simulink model "test_validation_gate"  (Simulink 7.6)
settings: Solver=FixedStepDiscrete  StartTime=0.0  StopTime=0  RelTol=1e-3
undefined symbols (not defined in the file): gray, Rec, Scale_Forward_B, Scale_Forward_G, Scale_Forward_H, Scale_Forward_R, Scale_Forward_S, Scale_Forward_V, SDTV
libraries: vipsnks x11, viptextngfix x2, vipconversions x2, vipsrcs x1, viptransforms x1
settings Model: Creator=Thing 1  LastModifiedBy=auvt
settings RTWCC: TargetLang=C++

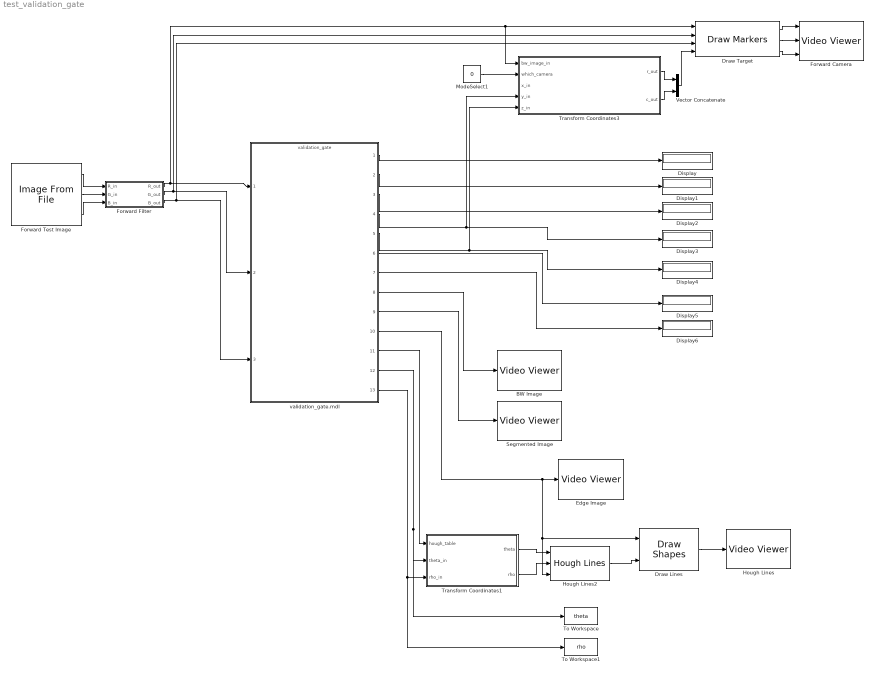
== system test_validation_gate ==
  BW Image : vipsnks/Video Viewer  DialogControllerArgs=DataTag1  inputType=Obsolete7b  imagePorts=One multidimensional signal  useColorMap=off  colormapValue=gray(256)  specRange=off  minInputVal=0  maxInputVal=255  FigPos=[651 667 290 272]  AxisZoom=on  trueSizedOnce=off  OpenAtMdlStart=on
  Display{,1..6} (7 alike) : Display
  Draw Lines : viptextngfix/Draw Shapes  DialogController=vipDDGCreate  DialogControllerArgs=DataTag2  shape=Lines  fill=off  fillClrSource=Specify via dialog  display=User-specified value  intensity=200  color=.5  opacity=0.6  viewport=Entire image  antialiasing=off  inType=Obsolete  imagePorts=One multidimensional signal  prodOutputMode=Binary point scaling  prodOutputWordLength=32  prodOutputFracLength=14  memoryMode=Specify word length  memoryWordLength=16  memoryFracLength=15  roundingMode=Floor  overflowMode=off
  Draw Target : viptextngfix/Draw Markers  DialogController=vipDDGCreate  DialogControllerArgs=DataTag3  shape=X-mark  size=7  fill=off  fillClrSource=Specify via dialog  display=User-specified value  intensity=200  color=[0 0 0]  opacity=0.6  viewport=Entire image  antialiasing=off  inType=Obsolete  imagePorts=Separate color signals  prodOutputMode=Binary point scaling  prodOutputWordLength=32  prodOutputFracLength=14  memoryMode=Specify word length  memoryWordLength=16  memoryFracLength=15  roundingMode=Floor  overflowMode=off
  Edge Image : vipsnks/Video Viewer  DialogControllerArgs=DataTag5  inputType=Obsolete7b  imagePorts=One multidimensional signal  useColorMap=off  colormapValue=gray(256)  specRange=off  minInputVal=0  maxInputVal=255  FigPos=[678 854 521 718]  AxisZoom=on  trueSizedOnce=off  OpenAtMdlStart=on
  Forward Camera : vipsnks/Video Viewer  DialogControllerArgs=DataTag7  inputType=Obsolete7b  imagePorts=Separate color signals  useColorMap=off  colormapValue=gray(256)  specRange=off  minInputVal=0  maxInputVal=255  FigPos=[1001 798 418 649]  AxisZoom=on  trueSizedOnce=off  OpenAtMdlStart=on
  Forward Filter : Subsystem
  Forward Test Image : vipsrcs/Image From File  Tag=vipblks_nd  DialogController=vipDDGCreate  DialogControllerArgs=DataTag20  SystemSampleTime=-1  FileName=/home/auvt/Desktop/Carlo/vlcsnap-2011-06-21-00h16m39s112.png  imagePorts=Separate color signals  Ts=-1  ImageDataType=double  Signed=on  WordLength=16  sdImageDataType=uint(8)  FractionLengthMode=User-defined  FractionLength=15  OutPortLabels=R|G|B
  Hough Lines : vipsnks/Video Viewer  DialogControllerArgs=DataTag22  inputType=Obsolete7b  imagePorts=One multidimensional signal  useColorMap=off  colormapValue=gray(256)  specRange=off  minInputVal=0  maxInputVal=255  FigPos=[-14 868 615 732]  AxisZoom=on  trueSizedOnce=off  OpenAtMdlStart=on
  Hough Lines2 : viptransforms/Hough Lines  DialogController=vipDDGCreate  DialogControllerArgs=DataTag23  sineCompMethod=Trigonometric function  thetaRes=pi/180  firstCoeffMode=Specify word length  firstCoeffWordLength=16  firstCoeffFracLength=15  prodOutputMode=Binary point scaling  prodOutputWordLength=32  prodOutputFracLength=16  roundingMode=Nearest  overflowMode=on
  ModeSelect1 : Constant  Value=0  SampleTime=-1
  Segmented Image : vipsnks/Video Viewer  DialogControllerArgs=DataTag25  inputType=Obsolete7b  imagePorts=One multidimensional signal  useColorMap=off  colormapValue=gray(256)  specRange=off  minInputVal=0  maxInputVal=255  FigPos=[645 429 251 293]  AxisZoom=on  trueSizedOnce=off  OpenAtMdlStart=on
  To Workspace : ToWorkspace  VariableName=theta  SampleTime=-1  SaveFormat=Array
  To Workspace1 : ToWorkspace  VariableName=rho  SampleTime=-1  SaveFormat=Array
  Transform Coordinates1 : Stateflow chart  TreatAsAtomicUnit=on  SystemSampleTime=[1/30 0]
  Transform Coordinates3 : Stateflow chart  TreatAsAtomicUnit=on  SystemSampleTime=[1/30 0]
  Vector Concatenate : Concatenate  Mode=Multidimensional array
  validation_gate.mdl : ModelReference  ModelNameDialog=validation_gate  SimulationMode=Accelerator  ModelReferenceVersion=1.1169  CopyOfModelName=validation_gate
  wires:
  Vector Concatenate/1 -> Draw Target/4
  Draw Target/2 -> Forward Camera/2
  Draw Target/1 -> Forward Camera/1
  Draw Target/3 -> Forward Camera/3
  ModeSelect1/1 -> Transform Coordinates3/2(which_camera)
  Transform Coordinates3/1(r_out) -> Vector Concatenate/1
  Transform Coordinates3/2(c_out) -> Vector Concatenate/2
  validation_gate.mdl/1 -> Display/1
  validation_gate.mdl/2 -> Display1/1
  validation_gate.mdl/3 -> Display2/1
  validation_gate.mdl/4 -> Display3/1, Transform Coordinates3/4(y_in)
  validation_gate.mdl/5 -> Display4/1, Transform Coordinates3/5(z_in)
  validation_gate.mdl/6 -> Display5/1
  validation_gate.mdl/7 -> Display6/1
  Forward Filter/1(R_out) -> validation_gate.mdl/1, Draw Target/1, Transform Coordinates3/1(bw_image_in)
  Forward Filter/2(G_out) -> validation_gate.mdl/2, Draw Target/2
  Forward Filter/3(B_out) -> validation_gate.mdl/3, Draw Target/3
  validation_gate.mdl/8 -> BW Image/1
  validation_gate.mdl/9 -> Segmented Image/1
  validation_gate.mdl/10 -> Edge Image/1, Hough Lines2/3, Draw Lines/1
  Forward Test Image/1 -> Forward Filter/1(R_in)
  Forward Test Image/2 -> Forward Filter/2(G_in)
  Forward Test Image/3 -> Forward Filter/3(B_in)
  validation_gate.mdl/11 -> Transform Coordinates1/1(hough_table)
  validation_gate.mdl/12 -> Transform Coordinates1/2(theta_in), To Workspace/1
  validation_gate.mdl/13 -> Transform Coordinates1/3(rho_in), To Workspace1/1
  Transform Coordinates1/1(theta) -> Hough Lines2/1
  Transform Coordinates1/2(rho) -> Hough Lines2/2
  Hough Lines2/1 -> Draw Lines/2
  Draw Lines/1 -> Hough Lines/1

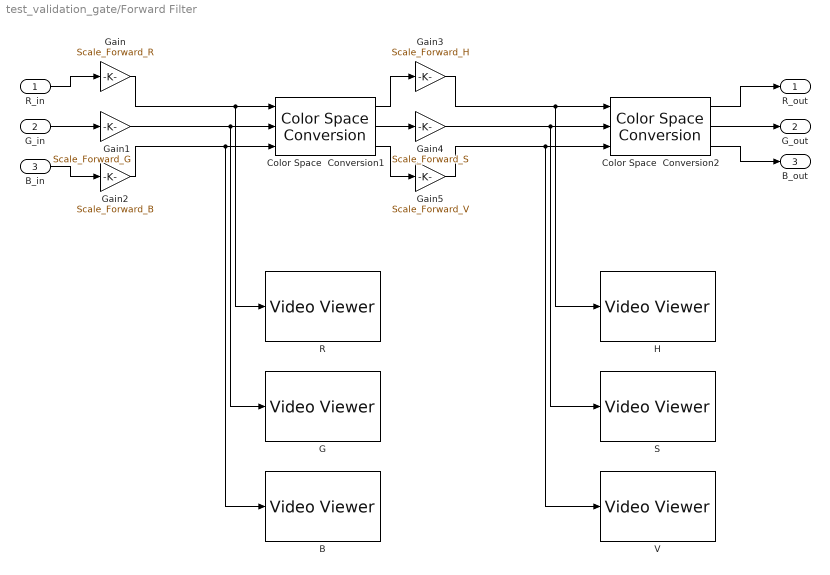
== system test_validation_gate/Forward Filter ==
  R_in : Inport  PortDimensions=Forward_Camera_Dimensions
  G_in : Inport  Port=2  PortDimensions=Forward_Camera_Dimensions
  B_in : Inport  Port=3  PortDimensions=Forward_Camera_Dimensions
  B : vipsnks/Video Viewer  DialogControllerArgs=DataTag9  inputType=Obsolete7b  imagePorts=One multidimensional signal  useColorMap=off  colormapValue=gray(256)  specRange=off  minInputVal=0  maxInputVal=255  FigPos=[-59 861 410 300]  AxisZoom=on  trueSizedOnce=off  OpenAtMdlStart=on
  Color Space  Conversion1 : vipconversions/Color Space  Conversion  conversion=Obsolete  conversionActive=R'G'B' to HSV  wp_str=D50  rec=Rec. 601 (SDTV)  sys=1125/60/2:1  imagePorts=Separate color signals
  Color Space  Conversion2 : vipconversions/Color Space  Conversion  conversion=Obsolete  conversionActive=HSV to R'G'B'  wp_str=D50  rec=Rec. 601 (SDTV)  sys=1125/60/2:1  imagePorts=Separate color signals
  G : vipsnks/Video Viewer  DialogControllerArgs=DataTag11  inputType=Obsolete7b  imagePorts=One multidimensional signal  useColorMap=off  colormapValue=gray(256)  specRange=off  minInputVal=0  maxInputVal=255  FigPos=[-76 583 410 300]  AxisZoom=on  trueSizedOnce=off  OpenAtMdlStart=on
  Gain : Gain  Gain=Scale_Forward_R
  Gain1 : Gain  Gain=Scale_Forward_G
  Gain2 : Gain  Gain=Scale_Forward_B
  Gain3 : Gain  Gain=Scale_Forward_H
  Gain4 : Gain  Gain=Scale_Forward_S
  Gain5 : Gain  Gain=Scale_Forward_V
  H : vipsnks/Video Viewer  DialogControllerArgs=DataTag13  inputType=Obsolete7b  imagePorts=One multidimensional signal  useColorMap=off  colormapValue=gray(256)  specRange=off  minInputVal=0  maxInputVal=255  FigPos=[262 436 410 300]  AxisZoom=on  trueSizedOnce=off  OpenAtMdlStart=on
  R : vipsnks/Video Viewer  DialogControllerArgs=DataTag15  inputType=Obsolete7b  imagePorts=One multidimensional signal  useColorMap=off  colormapValue=gray(256)  specRange=off  minInputVal=0  maxInputVal=255  FigPos=[-86 436 410 300]  AxisZoom=on  trueSizedOnce=off  OpenAtMdlStart=on
  S : vipsnks/Video Viewer  DialogControllerArgs=DataTag17  inputType=Obsolete7b  imagePorts=One multidimensional signal  useColorMap=off  colormapValue=gray(256)  specRange=off  minInputVal=0  maxInputVal=255  FigPos=[253 614 410 300]  AxisZoom=on  trueSizedOnce=off  OpenAtMdlStart=on
  V : vipsnks/Video Viewer  DialogControllerArgs=DataTag19  inputType=Obsolete7b  imagePorts=One multidimensional signal  useColorMap=off  colormapValue=gray(256)  specRange=off  minInputVal=0  maxInputVal=255  FigPos=[249 894 410 300]  AxisZoom=on  trueSizedOnce=off  OpenAtMdlStart=on
  R_out : Outport  OutDataTypeStr=double
  G_out : Outport  Port=2  OutDataTypeStr=double
  B_out : Outport  Port=3  OutDataTypeStr=double
  wires:
  R_in/1 -> Gain/1
  G_in/1 -> Gain1/1
  B_in/1 -> Gain2/1
  Gain/1 -> Color Space  Conversion1/1, R/1
  Gain1/1 -> Color Space  Conversion1/2, G/1
  Gain2/1 -> Color Space  Conversion1/3, B/1
  Color Space  Conversion1/1 -> Gain3/1
  Color Space  Conversion1/2 -> Gain4/1
  Color Space  Conversion1/3 -> Gain5/1
  Gain3/1 -> Color Space  Conversion2/1, H/1
  Gain4/1 -> Color Space  Conversion2/2, S/1
  Gain5/1 -> Color Space  Conversion2/3, V/1
  Color Space  Conversion2/1 -> R_out/1
  Color Space  Conversion2/2 -> G_out/1
  Color Space  Conversion2/3 -> B_out/1

== matlab function Transform Coordinates3 ==
  data: bw_image_in input double; which_camera input double; x_in input double; y_in input double; r_out output double; c_out output double; z_in input double
function [r_out, c_out] = transform_G2L(bw_image_in, which_camera, x_in, y_in, z_in)
% This function, "transform Global to Local coordinates," transforms
%   global coordinates that are sent to the controller into local
%   coordinates that can be displayed over images.
%
% 5-29-11
%
% Input
%   x_in, y_in, z_in = vectors of points in global (vehicle-centered)
%     coordinate system
%   bw_image_in = a 2-D array of pixel values (used only to extract image
%     size)
%   which_camera = selects which camera for relative coordinates
%                = 0 -> Forward camera
%                = 1 -> Down camera
%
% Output
%   r_out, c_out = row, column pairs in local coordinate system

[rows, cols] = size(bw_image_in);
if( which_camera == 0 )
    r_out = z_in + floor(rows/2);
    c_out = y_in + floor(cols/2);
else
    r_out = floor(rows/2) - x_in;
    c_out = y_in + floor(cols/2);
end

%{
if( which_camera == 0 )
    r_out = int32( z_in + floor(rows/2) );
    c_out = int32( y_in + floor(cols/2) );
else
    r_out = int32( floor(rows/2) - x_in );
    c_out = int32( y_in + floor(cols/2) );
end
%}
return

== matlab function Transform Coordinates1 ==
  data: hough_table input double; theta_in input double; rho_in input double; theta output double; rho output double
function [theta, rho] = draw_lines(hough_table, theta_in, rho_in)
%#eml

%{
len = min( length(rho_in), length(theta_in) );
rho = zeros(1, len);
theta = zeros(1, len);

for i = 1:len
    rho(i) = rho_in(i);
    theta(i) = theta_in(i);
end
%}



%% Initialize
% Only the (max_num_lines) with the most votes will be considered as
%   candidates for the validation gate
max_num_lines = 50;
[rho_length, theta_length] = size(hough_table);


% These vectors contain intermediate line information; as lines are
%   eliminated from these vectors, their values are set to zero
rho = zeros(1,max_num_lines);
theta = zeros(1,max_num_lines);


% Identify the most popular max_num_lines lines
i_index = ones(1,max_num_lines);
j_index = ones(1,max_num_lines);

m = 1;
while( m <= max_num_lines )
    
    max_votes = 0;
    for i = 1:rho_length
        for j = 1:theta_length
            if( hough_table(i,j) > max_votes )
                i_index(m) = i;
                j_index(m) = j;
                max_votes = hough_table(i,j);
            end
        end
    end
    
    rho(m) = rho_in(i_index(m));
    theta(m) = theta_in(j_index(m));
    hough_table(i_index(m),j_index(m)) = 0;
    m = m + 1;
    
end





return
